simulink model "DCMotor"  (R2021a)
settings: Solver=VariableStepAuto  StartTime=0.0  StopTime=10.0  RelTol=1e-3
libraries: slpidlib x1
settings Model: Creator=templ  LastModifiedBy=templ

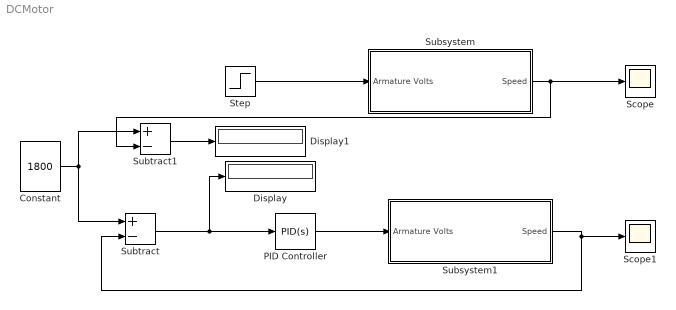
== system DCMotor ==
  Constant : Constant  Value=1800
  Display : Display
  Display1 : Display
  PID Controller : slpidlib/PID Controller  Controller=PID  Form=Parallel  TimeDomain=Continuous-time  UseExternalTs=off  SampleTime=-1  IntegratorMethod=Forward Euler  FilterMethod=Forward Euler  ControllerParametersSource=internal  P=0.0054833  I=0.04230  D=0.00017769  UseFilter=on  N=100  TunerSelectOption=Transfer Function Based (PID Tuner App)  InitialConditionSource=internal  InitialConditionForIntegrator=0  InitialConditionForFilter=0  DifferentiatorICPrevScaledInput=0  ExternalReset=none  TrackingMode=off  Kt=1  LimitOutput=off  SatLimitsSource=internal  UpperSaturationLimit=inf  LowerSaturationLimit=-inf  LinearizeAsGain=on  AntiWindupMode=none  Kb=1  POutMin=[]  POutMax=[]  IOutMin=[]  IOutMax=[]  DOutMin=[]  DOutMax=[]  NOutMin=[]  NOutMax=[]  SumOutMin=[]  SumOutMax=[]  SaturationOutMin=[]  SaturationOutMax=[]  PParamMin=[]  PParamMax=[]  IParamMin=[]  IParamMax=[]  DParamMin=[]  DParamMax=[]  NParamMin=[]  NParamMax=[]  KbParamMin=[]  KbParamMax=[]  KtParamMin=[]  KtParamMax=[]  KbOutMin=[]  KbOutMax=[]  KtOutMin=[]  KtOutMax=[]  IntegratorOutMin=[]  IntegratorOutMax=[]  FilterOutMin=[]  FilterOutMax=[]  SumI1OutMin=[]  SumI1OutMax=[]  SumI2OutMin=[]  SumI2OutMax=[]  SumI3OutMin=[]  SumI3OutMax=[]  SumI4OutMin=[]  SumI4OutMax=[]  SumDOutMin=[]  SumDOutMax=[]  DifferentiatorOutMin=[]  DifferentiatorOutMax=[]  FilterDiffOutCoefMin=[]  FilterDiffOutCoefMax=[]  ReciprocalOutMin=[]  ReciprocalOutMax=[]  SumDenOutMin=[]  SumDenOutMax=[]  SumNumOutMin=[]  SumNumOutMax=[]  DivideOutMin=[]  DivideOutMax=[]  UdiffTsProdOutMin=[]  UdiffTsProdOutMax=[]  NTsProdOutMin=[]  NTsProdOutMax=[]  UintegralTsProdOutMin=[]  UintegralTsProdOutMax=[]  UngainTsProdOutMin=[]  UngainTsProdOutMax=[]  IntegratorContinuousStateAttributes=''  IntegratorStateMustResolveToSignalObject=off  IntegratorRTWStateStorageClass=Auto  FilterContinuousStateAttributes=''  FilterStateMustResolveToSignalObject=off  FilterRTWStateStorageClass=Auto  ParallelPVariant=InternalParameters  IdealPVariant=Disabled  IVariant=InternalParameters  DVariant=InternalParameters  IntegratorVariant=Continuous  SatVariant=Disabled  AWVariant=Passthrough  PCopyVariant=Disabled  TRVariant=Disabled  FdbkBlocksVariant=Forward  IdealPFdbkVariant=Disabled  SatFdbkVariant=Disabled  DerivativeFilterVariant=ContFilter  NVariant=InternalParameters  NCopyVariant=Disabled  FilterICVariant=InternalICsFilter  IntegratorICVariant=InternalICs  ExternalResetVariant=Disabled  TRSumVariant=Passthrough  SumFdbkVariant=Disabled  SumVariant=Sum_PID  TsampFilterVariant=InternalTs  TsampNgainVariant=Passthrough  TsampIntegralVariant=Passthrough  ExternalSaturationOutDataTypeStr=Inherit: Same as second input
  Scope : Scope
  Scope1 : Scope
  Step : Step  After=12  SampleTime=0
  Subsystem : Subsystem
  Subsystem1 : Subsystem
  Subtract : Sum  Inputs=+-
  Subtract1 : Sum  Inputs=+-
  wires:
  Step/1 -> Subsystem/1(Armature Volts)
  Subsystem/1(Speed) -> Subtract1/2, Scope/1
  PID Controller/1 -> Subsystem1/1(Armature Volts)
  Constant/1 -> Subtract1/1, Subtract/1
  Subsystem1/1(Speed) -> Subtract/2, Scope1/1
  Subtract/1 -> Display/1, PID Controller/1
  Subtract1/1 -> Display1/1

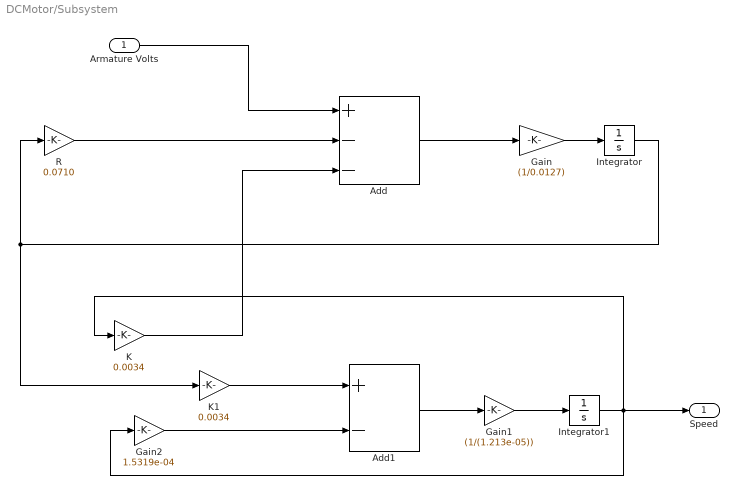
== system DCMotor/Subsystem ==
  Armature Volts : Inport
  Add : Sum  Inputs=+--
  Add1 : Sum  Inputs=+-
  Gain : Gain  Gain=(1/0.0127)
  Gain1 : Gain  Gain=(1/(1.213e-05))
  Gain2 : Gain  Gain=1.5319e-04
  Integrator : Integrator
  Integrator1 : Integrator
  K : Gain  Gain=0.0034
  K1 : Gain  Gain=0.0034
  R : Gain  Gain=0.0710
  Speed : Outport
  wires:
  Integrator1/1 -> Speed/1, K/1, Gain2/1
  Add/1 -> Gain/1
  Integrator/1 -> K1/1, R/1
  Gain2/1 -> Add1/2
  K/1 -> Add/3
  Armature Volts/1 -> Add/1
  R/1 -> Add/2
  Gain/1 -> Integrator/1
  Add1/1 -> Gain1/1
  K1/1 -> Add1/1
  Gain1/1 -> Integrator1/1

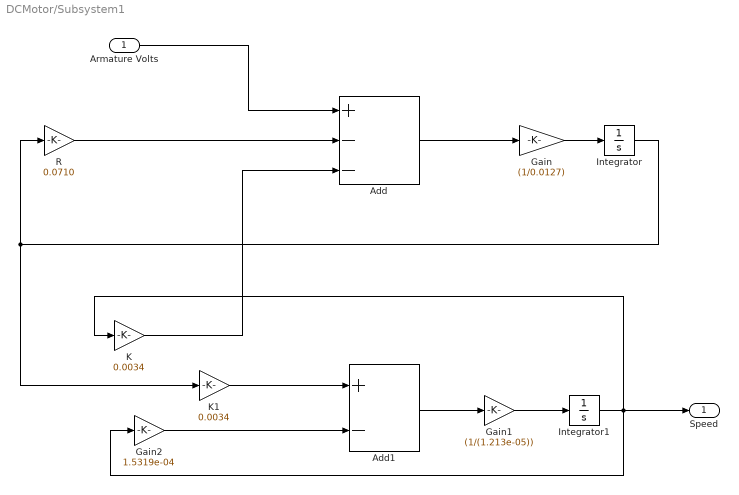
== system DCMotor/Subsystem1 ==
  Armature Volts : Inport
  Add : Sum  Inputs=+--
  Add1 : Sum  Inputs=+-
  Gain : Gain  Gain=(1/0.0127)
  Gain1 : Gain  Gain=(1/(1.213e-05))
  Gain2 : Gain  Gain=1.5319e-04
  Integrator : Integrator
  Integrator1 : Integrator
  K : Gain  Gain=0.0034
  K1 : Gain  Gain=0.0034
  R : Gain  Gain=0.0710
  Speed : Outport
  wires:
  Integrator1/1 -> Speed/1, K/1, Gain2/1
  Add/1 -> Gain/1
  Integrator/1 -> K1/1, R/1
  Gain2/1 -> Add1/2
  K/1 -> Add/3
  Armature Volts/1 -> Add/1
  R/1 -> Add/2
  Gain/1 -> Integrator/1
  Add1/1 -> Gain1/1
  K1/1 -> Add1/1
  Gain1/1 -> Integrator1/1
